simulink model "point_kinetic_equation"  (R2018b)
settings: Solver=VariableStepAuto  StartTime=0.0  StopTime=10.0  RelTol=1e-3
undefined symbols (not defined in the file): reactor
settings Model: Creator=tkdmc  LastModifiedBy=tkdmc

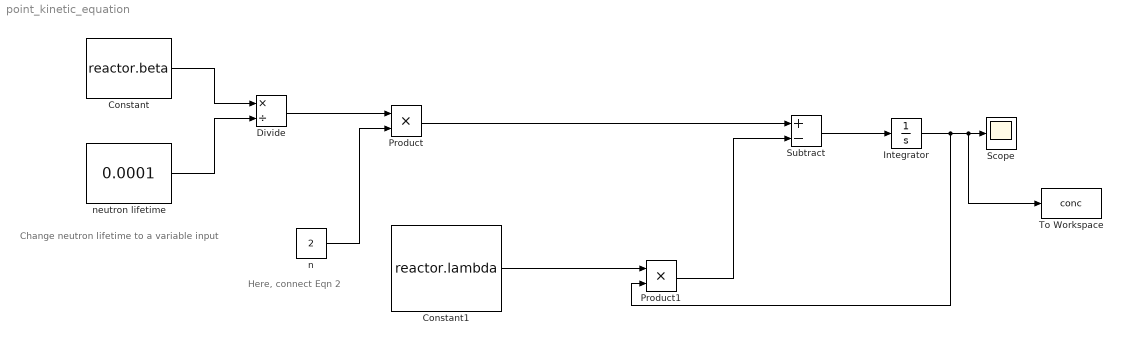
== system point_kinetic_equation ==
  note: Here, connect Eqn 2
  note: Change neutron lifetime to a variable input
  Constant : Constant  Value=reactor.beta
  Constant1 : Constant  Value=reactor.lambda
  Divide : Product  Inputs=*/
  Integrator : Integrator
  Product : Product
  Product1 : Product
  Scope : Scope
  Subtract : Sum  Inputs=+-
  To Workspace : ToWorkspace  VariableName=conc  SampleTime=-1
  "n " : Constant  Value=2
  neutron lifetime : Constant  Value=0.0001
  wires:
  Constant/1 -> Divide/1
  neutron lifetime/1 -> Divide/2
  Divide/1 -> Product/1
  "n "/1 -> Product/2
  Product/1 -> Subtract/1
  Constant1/1 -> Product1/1
  Product1/1 -> Subtract/2
  Subtract/1 -> Integrator/1
  Integrator/1 -> Product1/2, To Workspace/1, Scope/1
